simulink library "commnoisgen2"  (Simulink 6.0)
undefined symbols (not defined in the file or in its folder): m1, m2
libraries: dspsigattribs x4, simulink x4, dspbuff3 x3, commnoisgen2 x3, dspsrcs4 x2
settings Model: Creator=akansal  LastModifiedBy=fwei  ExtModeAutoUpdateStatusClock=off  ProdHWDeviceType=Specified

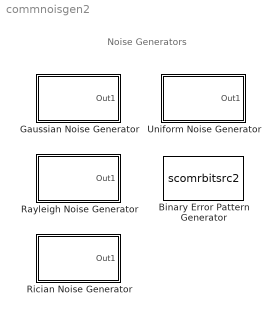
== system commnoisgen2 ==
  note: Noise Generators
  Binary Error Pattern Generator : S-Function  FunctionName=scomrbitsrc2  Parameters=n, prob, seed, Ts, frameBased, blksPerFrame, orient  mask(Binary Error Pattern Generator){n=7, prob=0.5, seed=12345, Ts=1, frameBased=off, blksPerFrame=1, orient=off}
      mask prompts: n "Block length:"; prob "Probabilities:"; seed "Initial seed:"; Ts "Sample time:"; frameBased "Frame-based outputs"; blksPerFrame "Blocks per frame:"; orient "Interpret vector parameters as 1-D"
      mask help: Generate a random binary vector with a limited number of ones. Use the "Probabilities" parameter to specify the probability that the output vector has a single one, two ones, three ones, etc. The sum of the elements in Probabilities must be less than or equal to one. One minus this sum is the probability that the output vector contains no ones.
      mask init:
      | eStr=commblkerrpatgen(gcb,'init');
      | if isequal(eStr.ecode1,1)  
      | 	error(eStr.emsg1);
      | elseif isequal(eStr.ecode2,1),
      | 	error(eStr.emsg2);
      | end
      mask Help: helpview(commbhelp);
      mask CallbackString: ||||commblkerrpatgen(gcb,'cbFrameBased');||commblkerrpatgen(gcb,'cbOrient');
      mask Display:
      | plot(0,0,100,100,[95 5 10 10 10 reshape(([85*[0:1/15:1-1/15]+10; 85*[1/15:1/15:1]+10]),1,30)],[75 75 75 70 95 reshape([randsrc(1,15,[80,90],12345); randsrc(1,15,[80,90],12345)],1,30)]);
      | disp('Error Pattern');
  Gaussian Noise Generator : Subsystem  mask(Gaussian Noise Generator){m=0, d=1, s=41, Ts=1, frameBased=off, sampPerFrame=1, orient=off}
      mask prompts: m "Mean value:"; d "Variance (vector or matrix):"; s "Initial seed:"; Ts "Sample time:"; frameBased "Frame-based outputs"; sampPerFrame "Samples per frame:"; orient "Interpret vector parameters as 1-D"
      mask help: Generate Gaussian distributed noise with given mean and variance values.
      mask init:
      | if isnumeric(d) & isequal(size(d),[1,1]), d=d*ones(1,max(length(m),length(s)));end
      | if(frameBased & sampPerFrame > 1),
      |   buffic=commblkgaussiansrc2(gcb,'UpdateIc',{m,d,s}); end;
      | [m,d,s,eStr]=commblkgaussiansrc2(gcb,'init',{m,d,s});
      | if(eStr.ecode==1)
      |     error(eStr.emsg);
      | end;
      mask Help: helpview(commbhelp)
      mask CallbackString: ||||commblkgaussiansrc2(gcb,'cbFrameBased');||commblkgaussiansrc2(gcb,'cbOrient');
      mask Display:
      | plot(0,0,100,100,[95 5 10 10 10 (100-15)*[0:1/30:1]+10],[75 75 75 70 95 70    58 76 77 63 86 86 74 78 76 73 82 69 96 73 76 85 75 74 66 77 61 82 91 68    83 87 59 60 80 71]);
      | disp('\nGaussian')
  Rayleigh Noise Generator : Subsystem  mask(Rayleigh Noise Generator){alpha=1, seed=47, Ts=1, frameBased=off, sampPerFrame=1, orient=off}
      mask prompts: alpha "Sigma:"; seed "Initial seed:"; Ts "Sample time:"; frameBased "Frame-based outputs"; sampPerFrame "Samples per frame:"; orient "Interpret vector parameters as 1-D"
      mask help: Generate Rayleigh distributed noise.The output vector size of this block is the same as the vector size of the seed.
      mask init:
      | if(frameBased & sampPerFrame > 1)
      |    buffic = commblkrayleighsrc2(gcb,'UpdateIc',{alpha,seed});end;
      | [alpha,seed,eStr]=commblkrayleighsrc2(gcb,'init',{alpha,seed});
      | if(eStr.ecode==1)
      |     error(eStr.emsg);
      | end;
      mask Help: helpview(commbhelp)
      mask CallbackString: |||commblkrayleighsrc2(gcb,'cbFrameBased');||commblkrayleighsrc2(gcb,'cbOrient');
      mask Display: plot(0,0,100,100,[95 5 10 10 10 (100-15)*[0:1/30:1]+10],[75 75 75 70 95 91    87 91 88 81 80 81 85 89 81 91 86 82 89 85 83 88 87 90 94 85 92 78 94 80    80 92 89 77 75 92]);disp('Rayleigh')
  Rician Noise Generator : Subsystem  mask(Rician Noise Generator){specMethod=K-factor, iMean=sqrt(2), qMean=sqrt(2), K=2, s=1, seed=59, Ts=1, frameBased=off, sampPerFrame=1, orient=off}
      mask prompts: specMethod "Specification method:"; iMean "In phase component (mean):"; qMean "Quadrature component (mean):"; K "Rician K-factor:"; s "Sigma:"; seed "Initial seed:"; Ts "Sample time:"; frameBased "Frame-based outputs"; sampPerFrame "Samples per frame:"; orient "Interpret vector parameters as 1-D"
      mask help: Generate Rician distributed noise. The output vector size of this block is the same as the vector size of the seed.
      mask init:
      | if(frameBased & sampPerFrame > 1)
      | buffic=commblkriciansrc2(gcb,'UpdateIc',{iMean, qMean, K, s});end;
      | [m1, m2, eStr]=commblkriciansrc2(gcb,'init',{iMean, qMean, K, s});
      | if(eStr.ecode==1)
      |     error(eStr.emsg);
      | end;
      mask Help: helpview(commbhelp)
      mask StyleString: popup(K-factor|Quadrature components),edit,edit,edit,edit,edit,edit,checkbox,edit,checkbox
      mask CallbackString: commblkriciansrc2(gcb,'SpecMethod');|||||||commblkriciansrc2(gcb,'cbFrameBased');||commblkriciansrc2(gcb,'cbOrient');
      mask Display:
      | plot(0,0,100,100,[95 5 10 10 10 (100-15)*[0:1/30:1]+10],[75 75 75 70 95 90    94 94 90 83 84 79 87 81 94 89 83 89 80 83 93 88 79 91 87 77 79 87 87 82    86 84 75 75 81 75]);
      | disp('Rician');
  Uniform Noise Generator : Subsystem  mask(Uniform Noise Generator){low=0, up=1, seed=31, Ts=1, frameBased=off, sampPerFrame=1, orient=off}
      mask prompts: low "Noise lower bound:"; up "Noise upper bound:"; seed "Initial seed:"; Ts "Sample time:"; frameBased "Frame-based outputs"; sampPerFrame "Samples per frame:"; orient "Interpret vector parameters as 1-D"
      mask help: Generate uniformly distributed noise between the upper and lower bounds.
      mask init:
      | eStr=commblkuniformsrc2(gcb,'init');
      | if(eStr.ecode==1)
      |     error(eStr.emsg);
      | end
      mask Help: helpview(commbhelp)
      mask CallbackString: ||||commblkuniformsrc2(gcb,'cbFrameBased');||commblkuniformsrc2(gcb,'cbOrient');
      mask Display: plot(0,0,100,100,[95 5 10 10 10 (100-15)*[0:1/30:1]+10],[75 75 75 70 95  94  79 87 84 92 90 84 75 91 83 87 90 93 89 78 83 93 93 83 92 76 82 91 75 77    79 78 87 80 78 75]);disp('Uniform')

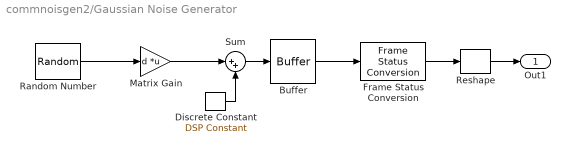
== system commnoisgen2/Gaussian Noise Generator ==
  Buffer : dspbuff3/Buffer  N=1  V=0  ic=0
  Discrete Constant : dspsrcs4/DSP Constant  Value=m  SampleMode=Discrete  discreteOutput=Sample-based (interpret vectors as 1-D)  continuousOutput=Sample-based  sampTime=Ts  framePeriod=Ts  dataType=Inherit from 'Constant value'  wordLen=16  udDataType=sfix(16)  fracBitsMode=Best precision  numFracBits=15  InterpretAs1D=on  Ts=Ts  FramebasedOutput=off
  Frame Status Conversion : dspsigattribs/Frame Status Conversion  growRefPort=off  outframe=Sample-based
  Matrix Gain : Gain  Gain=d  Multiplication=Matrix(K*u)
  Random Number : RandomNumber  Seed=s  SampleTime=Ts
  Reshape : simulink/Math Operations/Reshape  OutputDimensionality=1-D array  OutputDimensions=[sampPerFrame,length(s)]
  Sum : Sum  Inputs=|++  SaturateOnIntegerOverflow=on  InputSameDT=on
  Out1 : Outport  InitialOutput=0
  wires:
  Discrete Constant/1 -> Sum/2
  Reshape/1 -> Out1/1
  Buffer/1 -> Frame Status Conversion/1
  Frame Status Conversion/1 -> Reshape/1
  Matrix Gain/1 -> Sum/1
  Random Number/1 -> Matrix Gain/1
  Sum/1 -> Buffer/1

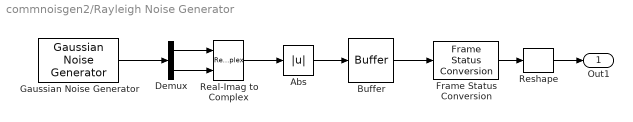
== system commnoisgen2/Rayleigh Noise Generator ==
  Abs : Abs  SaturateOnIntegerOverflow=on
  Buffer : dspbuff3/Buffer  N=1  V=0  ic=0
  Demux : Demux  Outputs=2
  Frame Status Conversion : dspsigattribs/Frame Status Conversion  growRefPort=off  outframe=Sample-based
  Gaussian Noise Generator : commnoisgen2/Gaussian Noise Generator  m=0  d=alpha  s=seed  Ts=Ts  frameBased=off  sampPerFrame=1  orient=on
  Real-Imag to Complex : RealImagToComplex
  Reshape : simulink/Math Operations/Reshape  OutputDimensionality=1-D array  OutputDimensions=[1,length(seed)]
  Out1 : Outport
  wires:
  Buffer/1 -> Frame Status Conversion/1
  Frame Status Conversion/1 -> Reshape/1
  Reshape/1 -> Out1/1
  Real-Imag to Complex/1 -> Abs/1
  Demux/2 -> Real-Imag to Complex/2
  Demux/1 -> Real-Imag to Complex/1
  Gaussian Noise Generator/1 -> Demux/1
  Abs/1 -> Buffer/1

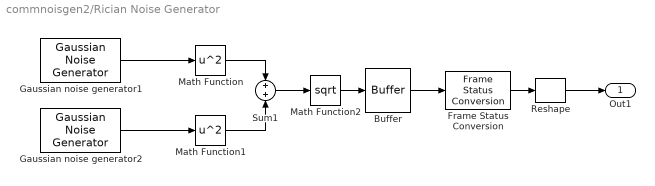
== system commnoisgen2/Rician Noise Generator ==
  Buffer : dspbuff3/Buffer  N=1  V=0  ic=0
  Frame Status Conversion : dspsigattribs/Frame Status Conversion  growRefPort=off  outframe=Sample-based
  Gaussian noise generator1 : commnoisgen2/Gaussian Noise Generator  m=m1  d=s.^2  s=seed  Ts=Ts  frameBased=off  sampPerFrame=1  orient=off
  Gaussian noise generator2 : commnoisgen2/Gaussian Noise Generator  m=m2  d=s.^2  s=seed+max(seed)  Ts=Ts  frameBased=off  sampPerFrame=1  orient=off
  Math Function : Math  Operator=square  SaturateOnIntegerOverflow=on
  Math Function1 : Math  Operator=square  SaturateOnIntegerOverflow=on
  Math Function2 : Math  Operator=sqrt  SaturateOnIntegerOverflow=on
  Reshape : simulink/Math Operations/Reshape  OutputDimensionality=1-D array  OutputDimensions=[1,length(seed)]
  Sum1 : Sum  SaturateOnIntegerOverflow=on  InputSameDT=on
  Out1 : Outport
  wires:
  Buffer/1 -> Frame Status Conversion/1
  Frame Status Conversion/1 -> Reshape/1
  Reshape/1 -> Out1/1
  Math Function2/1 -> Buffer/1
  Math Function1/1 -> Sum1/2
  Math Function/1 -> Sum1/1
  Sum1/1 -> Math Function2/1
  Gaussian noise generator2/1 -> Math Function1/1
  Gaussian noise generator1/1 -> Math Function/1

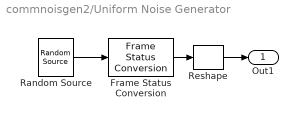
== system commnoisgen2/Uniform Noise Generator ==
  Frame Status Conversion : dspsigattribs/Frame Status Conversion  growRefPort=off  outframe=Sample-based
  Random Source : dspsrcs4/Random Source  SrcType=Uniform  NormMethod=Ziggurat  CltLength=12  Min=low  Max=up  Mean=0  Var=1  RepMode=Specify seed  Seed=seed  Inherit=off  SampMode=Discrete  SampTime=Ts  SampFrame=1  DataType=Double  OutComplex=Real
  Reshape : simulink/Math Operations/Reshape  OutputDimensionality=1-D array  OutputDimensions=[sampPerFrame,max([length(low),length(up),length(seed)])]
  Out1 : Outport
  wires:
  Frame Status Conversion/1 -> Reshape/1
  Reshape/1 -> Out1/1
  Random Source/1 -> Frame Status Conversion/1
